simulink model "PR"  (R2022a)
settings: Solver=FixedStepDiscrete  StartTime=0.0  StopTime=0.5  FixedStep=Ts_Power  RelTol=1e-3
InitFcn:
  | clc;
  | %clear;
  | 
  | %%simulation paremeter
  | fsw = 20e3;%switch freq
  | Ts_Control = 1/fsw;%control period
  | Ts_Power = 1 / fsw/64;%simulation step
  | Ts_Sample = 1 / fsw;%sample period
  | Tscon = Ts_Control;
  | %%system parameter
  | L = 250e-6;
  | L1 = L;
  | L2 = L;
  | C = 620e-6;
  | R = 75;
  | Uc_init = 390;%capacitor voltage init
  | v_ref = 390;
  | 
  | %%controller parameter
  | k_cp=-0.0235;
  | k_ci=-1.871e3;
  | 
  | k_vi = 1.7714;
  | k_vp = 0.0488;
undefined symbols (not defined in the file or in its folder): DiscIntNeverNeededParam
libraries: spspowerguiLib x1
settings Model: Creator=xg  LastModifiedBy=12586
settings SolverCC: AlgebraicLoopSolver=TrustRegion
settings DataIOCC: ReturnWorkspaceOutputs=off
settings DebuggingCC: ArithmeticOperatorsInVariantConditions=warning
settings SFSimCC: CustomCodeUndefinedFunction=UseInterfaceOnly

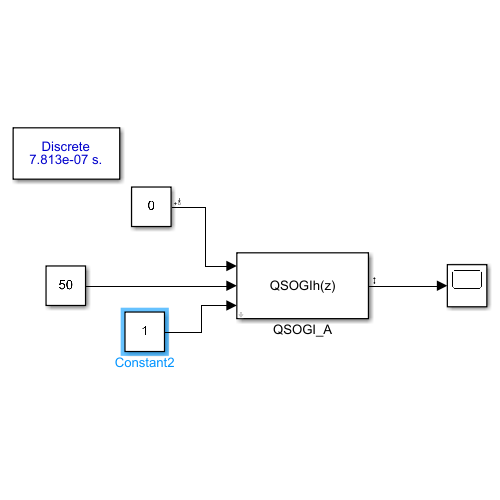
[thumbnail: Simulink's stored preview of the top-level diagram]
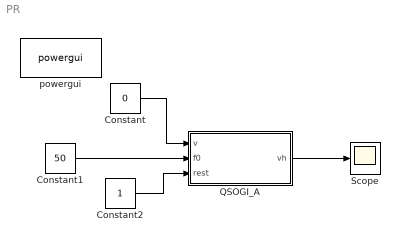
== system PR ==
  Constant : Constant  Value=0  SampleTime=1/20e3
  Constant1 : Constant  Value=50  SampleTime=1/20e3
  Constant2 : Constant  SampleTime=1/20e3
  QSOGI_A : Subsystem  mask{h=1, KIh=-86, wc=0.002, phch=0.0036, Ts=Ts_Control}
      mask prompts: h "Selected harmonic orders"; KIh "Integral gain of QSOGI"; wc "Inversion of maximum gain"; phch "Phase compensation angle"; Ts "Sampling Period"
      mask Display: disp('QSOGIh(z)')
  Scope : Scope
  powergui : spspowerguiLib/powergui  Priority=1  SimulationMode=Discrete  SampleTime=Ts_Power  frequency=60  Iterations=50  frequencyindice=0  Pbase=100e6  ErrMax=1e-4  UnitsV=kV  UnitsW=MW  buscounter=0  FunctionMessages=off  echomessages=off  EnableUseOfTLC=off  CurrentSourceSwitches=off  DisableSnubberDevices=off  DisableRonSwitches=off  DisableVfSwitches=off  DisplayEquations=off  AutomaticDiscreteSolvers=off  SolverType=Tustin/Backward Euler (TBE)  Interpol=off  ExternalGateDelay=off  methode=off  Ts=100  x0status=blocks  SPID=on  SwTol=0  HookPort=off  NonlinearTolerance=1e-4  nMaxIteration=100  ContinueOnMaxIteration=off  RestoreLinks=warning  ResistiveCurrentMeasurement=off  Frange=[0:2:500]  Ylog=off  Xlog=on  ShowGrid=off  save=off  variable=ZData  structure=logsout  ZoomFFT=on  StartTime=0.5  cycles=1  DisplayStyle=1  fundamental=50  FreqAxis=off  MaxFrequency=30000  frequencyindicesteady=1  RmsSteady=1  display=off
  wires:
  Constant/1 -> QSOGI_A/1(v)
  Constant1/1 -> QSOGI_A/2(f0)
  Constant2/1 -> QSOGI_A/3(rest)
  QSOGI_A/1(vh) -> Scope/1

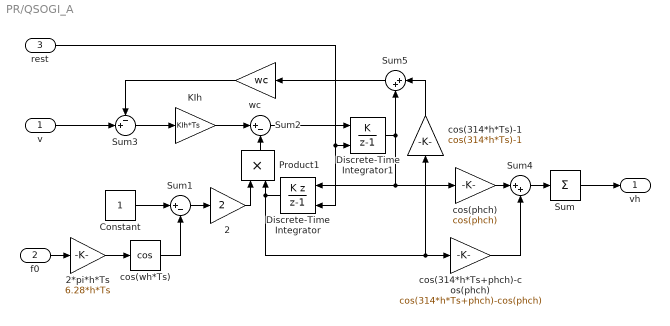
== system PR/QSOGI_A ==
  v : Inport
  f0 : Inport  Port=2
  rest : Inport  Port=3
  2 : Gain  Gain=2
  2*pi*h*Ts : Gain  Gain=6.28*h*Ts
  Constant : Constant  SampleTime=Tscon
  Discrete-Time Integrator : DiscreteIntegrator  IntegratorMethod=Accumulation: Backward Euler  ExternalReset=level  SampleTime=-1  ICPrevOutput=DiscIntNeverNeededParam  ICPrevScaledInput=DiscIntNeverNeededParam
  Discrete-Time Integrator1 : DiscreteIntegrator  IntegratorMethod=Accumulation: Forward Euler  ExternalReset=level  SampleTime=-1  ICPrevOutput=DiscIntNeverNeededParam  ICPrevScaledInput=DiscIntNeverNeededParam
  KIh : Gain  Gain=KIh*Ts
  Product1 : Product
  Sum : Sum  Inputs=+
  Sum1 : Sum  Inputs=|+-
  Sum2 : Sum  Inputs=|+-
  Sum3 : Sum  Inputs=-+|
  Sum4 : Sum  Inputs=|++
  Sum5 : Sum  Inputs=|++
  cos(314*h*Ts)-1 : Gain  Gain=cos(314*h*Ts)-1
  cos(314*h*Ts+phch)-cos(phch) : Gain  Gain=cos(314*h*Ts+phch)-cos(phch)
  cos(phch) : Gain  Gain=cos(phch)
  cos(wh*Ts) : Trigonometry  Operator=cos
  wc : Gain  Gain=wc
  vh : Outport  VectorParamsAs1DForOutWhenUnconnected=off
  wires:
  rest/1 -> Discrete-Time Integrator1/2, Discrete-Time Integrator/2
  Product1/1 -> Sum2/2
  Sum2/1 -> Discrete-Time Integrator1/1
  v/1 -> Sum3/2
  KIh/1 -> Sum2/1
  f0/1 -> 2*pi*h*Ts/1
  Discrete-Time Integrator1/1 -> Discrete-Time Integrator/1, cos(phch)/1, Sum5/2
  Discrete-Time Integrator/1 -> cos(314*h*Ts)-1/1, cos(314*h*Ts+phch)-cos(phch)/1, Product1/2
  Sum4/1 -> Sum/1
  2*pi*h*Ts/1 -> cos(wh*Ts)/1
  cos(wh*Ts)/1 -> Sum1/2
  Constant/1 -> Sum1/1
  Sum1/1 -> 2/1
  2/1 -> Product1/1
  cos(phch)/1 -> Sum4/1
  cos(314*h*Ts+phch)-cos(phch)/1 -> Sum4/2
  Sum/1 -> vh/1
  wc/1 -> Sum3/1
  Sum3/1 -> KIh/1
  Sum5/1 -> wc/1
  cos(314*h*Ts)-1/1 -> Sum5/1
